simulink model "HANcoder_E407_GTSync_v5"  (R2018b)
settings: Solver=FixedStepDiscrete  StartTime=0.0  StopTime=1  FixedStep=0.01  RelTol=1e-3
PreLoadFcn:
  | librarySetup
  | eval([bdroot,'_startup']) %Calling [modelName]_startup.m
values from neighbouring files (symbols this model uses):
  basic_cycle_duration = TM_Reset_Board + COMP_duration    (= 170)    [HANcoder_E407_GTSync_v5_startup.m]
  comm_delay_estimation1 = round(comm_delay_measured*hardware_granularity/frequency_IRQ)    [HANcoder_E407_GTSync_v5_startup.m]
  comm_delay_estimation2 = round(comm_delay_measured*hardware_granularity/frequency_IRQ)    [HANcoder_E407_GTSync_v5_startup.m]
  COMM_Period = 25    [HANcoder_E407_GTSync_v5_startup.m]
  COMM_Phase1 = floor(COMM_Period/5)    [HANcoder_E407_GTSync_v5_startup.m]
  COMM_Phase2 = floor(4*COMM_Period/5)    [HANcoder_E407_GTSync_v5_startup.m]
  frequency_IRQ = 100    [HANcoder_E407_GTSync_v5_startup.m]
  HANtuneOverride = Simulink.Parameter    [HANcoder_E407_GTSync_v5_startup.m]
  idle_time_init = basic_cycle_duration*matrix_rows    (= 340)    [HANcoder_E407_GTSync_v5_startup.m]
  LED_ticks_toggle = 10000    [HANcoder_E407_GTSync_v5_startup.m]
  Master_Role = 1    [HANcoder_E407_GTSync_v5_startup.m]
  matrix_rows = 2    [HANcoder_E407_GTSync_v5_startup.m]
  MEX_Flag = 0    [HANcoder_E407_GTSync_v5_startup.m]
  Slave_Role = 2    [HANcoder_E407_GTSync_v5_startup.m]
  Sync_ID = 1    [HANcoder_E407_GTSync_v5_startup.m]
  TM_Check_Sync = TM_COMM_Sync   + COMM_duration    (= 30)    [HANcoder_E407_GTSync_v5_startup.m]
  TM_Check_TOuts = TM_Count_Vote3 + COMP_duration    (= 150)    [HANcoder_E407_GTSync_v5_startup.m]
  TM_Check_Vote1 = TM_COMM_Vote1  + COMM_duration    (= 70)    [HANcoder_E407_GTSync_v5_startup.m]
  TM_Check_Vote2 = TM_COMM_Vote2  + COMM_duration    (= 105)    [HANcoder_E407_GTSync_v5_startup.m]
  TM_Check_Vote3 = TM_COMM_Vote3  + COMM_duration    (= 140)    [HANcoder_E407_GTSync_v5_startup.m]
  TM_COMM_Sync = basic_cycle_start    (= 5)    [HANcoder_E407_GTSync_v5_startup.m]
  TM_COMM_Vote1 = TM_Vote_Dec    + COMP_duration    (= 45)    [HANcoder_E407_GTSync_v5_startup.m]
  TM_COMM_Vote2 = TM_Count_Vote1 + COMP_duration    (= 80)    [HANcoder_E407_GTSync_v5_startup.m]
  TM_COMM_Vote3 = TM_Count_Vote2 + COMP_duration    (= 115)    [HANcoder_E407_GTSync_v5_startup.m]
  TM_Count_Vote1 = TM_Check_Vote1 + COMP_duration    (= 75)    [HANcoder_E407_GTSync_v5_startup.m]
  TM_Count_Vote2 = TM_Check_Vote2 + COMP_duration    (= 110)    [HANcoder_E407_GTSync_v5_startup.m]
  TM_Count_Vote3 = TM_Check_Vote3 + COMP_duration    (= 145)    [HANcoder_E407_GTSync_v5_startup.m]
  TM_New_Master = TM_Check_TOuts + COMP_duration    (= 155)    [HANcoder_E407_GTSync_v5_startup.m]
  TM_Reset_Board = TM_Reset_Var   + COMP_duration    (= 165)    [HANcoder_E407_GTSync_v5_startup.m]
  TM_Reset_Var = TM_New_Master  + COMP_duration    (= 160)    [HANcoder_E407_GTSync_v5_startup.m]
  TM_Update_LT = TM_Check_Sync  + COMP_duration    (= 35)    [HANcoder_E407_GTSync_v5_startup.m]
  TM_Vote_Dec = TM_Update_LT   + COMP_duration    (= 40)    [HANcoder_E407_GTSync_v5_startup.m]
  Toggle_Flag = 1    [HANcoder_E407_GTSync_v5_startup.m]
  Vote1_ID = 12    [HANcoder_E407_GTSync_v5_startup.m]
  Vote2_ID = 22    [HANcoder_E407_GTSync_v5_startup.m]
  Vote3_ID = 32    [HANcoder_E407_GTSync_v5_startup.m]
undefined symbols (not defined in the file or in its folder): A0, A1, A2, A3, CON2
libraries: HANcoder_STM32_Target x25, hdlsllib x21, simulink x3, simulink_extras x1
(part 7 of 7)

== system HANcoder_E407_GTSync_v5/HANcoder STM32 Target - E407-STM32 algorithm/Global Ticks Increment/CAN Management/Matrix Cycle Manager/COMP Task - Rx_Vote2_Check/Process_Messages1/Demux message CAN1 and check coherence ==
  CAN1_Rx_msg : Inport  OutDataTypeStr=Bus: msg_buffer_type
  expected_local_time : Inport  Port=2
  expected_basic_cycle : Inport  Port=3
  Enable : EnablePort
  AND : Logic  IconShape=distinctive  AllPortsSameDT=off  OutDataTypeStr=boolean
  Bus Creator : BusCreator  Inputs=3  OutDataTypeStr=Bus: demux_msg_buffer_type
  Bus Selector : BusSelector  OutputSignals=Buffer_1,Buffer_2,Buffer_3,Buffer_4,Buffer_5,Buffer_6,Buffer_7,Buffer_8
  Equal : RelationalOperator  Operator===  OutDataTypeStr=boolean  RndMeth=Simplest
  Equal2 : RelationalOperator  Operator===  OutDataTypeStr=boolean  RndMeth=Simplest
  Terminator{3..4,6..7} (4 alike) : Terminator
  UINT8 to UINT16 : Subsystem
  CAN1_msg : Outport  OutDataTypeStr=Bus: demux_msg_buffer_type
  CAN1_msg_coherent : Outport  Port=2  OutputWhenDisabled=reset  InitialOutput=0
  wires:
  Bus Selector/2 -> UINT8 to UINT16/1(In1)  "<Buffer_2>"
  UINT8 to UINT16/1(Out1) -> Bus Creator/2, Equal/1
  Bus Selector/1 -> Bus Creator/1  "<Buffer_1>"
  Bus Selector/4 -> Bus Creator/3, Equal2/1  "<Buffer_4>"
  Bus Selector/3 -> UINT8 to UINT16/2(In2)  "<Buffer_3>"
  CAN1_Rx_msg/1 -> Bus Selector/1
  Equal2/1 -> AND/2
  Equal/1 -> AND/1
  AND/1 -> CAN1_msg_coherent/1
  expected_local_time/1 -> Equal/2
  expected_basic_cycle/1 -> Equal2/2
  Bus Creator/1 -> CAN1_msg/1
  Bus Selector/6 -> Terminator3/1  "<Buffer_6>"
  Bus Selector/5 -> Terminator4/1  "<Buffer_5>"
  Bus Selector/7 -> Terminator6/1  "<Buffer_7>"
  Bus Selector/8 -> Terminator7/1  "<Buffer_8>"

== system HANcoder_E407_GTSync_v5/HANcoder STM32 Target - E407-STM32 algorithm/Global Ticks Increment/CAN Management/Matrix Cycle Manager/COMP Task - Rx_Vote2_Check/Process_Messages1/Demux message CAN2 and check coherence ==
  CAN2_Rx_msg : Inport  OutDataTypeStr=Bus: msg_buffer_type
  expected_local_time : Inport  Port=2
  expected_basic_cycle : Inport  Port=3
  Enable : EnablePort
  AND : Logic  IconShape=distinctive  AllPortsSameDT=off  OutDataTypeStr=boolean
  Bus Creator : BusCreator  Inputs=3  OutDataTypeStr=Bus: demux_msg_buffer_type
  Bus Selector : BusSelector  OutputSignals=Buffer_1,Buffer_2,Buffer_3,Buffer_4,Buffer_5,Buffer_6,Buffer_7,Buffer_8
  Equal : RelationalOperator  Operator===  OutDataTypeStr=boolean  RndMeth=Simplest
  Equal2 : RelationalOperator  Operator===  OutDataTypeStr=boolean  RndMeth=Simplest
  Terminator{3..4,6..7} (4 alike) : Terminator
  UINT8 to UINT16 : Subsystem
  CAN2_msg_coherent : Outport  OutputWhenDisabled=reset  InitialOutput=0
  CAN2_msg : Outport  Port=2  OutDataTypeStr=Bus: demux_msg_buffer_type
  wires:
  Bus Selector/2 -> UINT8 to UINT16/1(In1)  "<Buffer_2>"
  UINT8 to UINT16/1(Out1) -> Bus Creator/2, Equal/1
  Bus Selector/1 -> Bus Creator/1  "<Buffer_1>"
  Bus Selector/4 -> Bus Creator/3, Equal2/1  "<Buffer_4>"
  Bus Selector/3 -> UINT8 to UINT16/2(In2)  "<Buffer_3>"
  CAN2_Rx_msg/1 -> Bus Selector/1
  Equal/1 -> AND/1  "expected_lt_Vote2_CAN2_s"
  AND/1 -> CAN2_msg_coherent/1
  expected_local_time/1 -> Equal/2
  expected_basic_cycle/1 -> Equal2/2
  Bus Creator/1 -> CAN2_msg/1
  Bus Selector/6 -> Terminator3/1  "<Buffer_6>"
  Bus Selector/5 -> Terminator4/1  "<Buffer_5>"
  Bus Selector/7 -> Terminator6/1  "<Buffer_7>"
  Bus Selector/8 -> Terminator7/1  "<Buffer_8>"
  Equal2/1 -> AND/2  "expected_bc_Vote2_CAN2_s"

== system HANcoder_E407_GTSync_v5/HANcoder STM32 Target - E407-STM32 algorithm/Global Ticks Increment/CAN Management/Matrix Cycle Manager/COMP Task - Rx_Vote3_Check/Process_Messages1/Demux message CAN1 and check coherence ==
  CAN1_Rx_msg : Inport  OutDataTypeStr=Bus: msg_buffer_type
  expected_local_time : Inport  Port=2
  expected_basic_cycle : Inport  Port=3
  Enable : EnablePort
  AND : Logic  IconShape=distinctive  AllPortsSameDT=off  OutDataTypeStr=boolean
  Bus Creator : BusCreator  Inputs=3  OutDataTypeStr=Bus: demux_msg_buffer_type
  Bus Selector : BusSelector  OutputSignals=Buffer_1,Buffer_2,Buffer_3,Buffer_4,Buffer_5,Buffer_6,Buffer_7,Buffer_8
  Equal : RelationalOperator  Operator===  OutDataTypeStr=boolean  RndMeth=Simplest
  Equal2 : RelationalOperator  Operator===  OutDataTypeStr=boolean  RndMeth=Simplest
  Terminator{3..4,6..7} (4 alike) : Terminator
  UINT8 to UINT16 : Subsystem
  CAN1_msg : Outport  OutDataTypeStr=Bus: demux_msg_buffer_type
  CAN1_msg_coherent : Outport  Port=2  OutputWhenDisabled=reset  InitialOutput=0
  wires:
  Bus Selector/2 -> UINT8 to UINT16/1(In1)  "<Buffer_2>"
  UINT8 to UINT16/1(Out1) -> Bus Creator/2, Equal/1
  Bus Selector/1 -> Bus Creator/1  "<Buffer_1>"
  Bus Selector/4 -> Bus Creator/3, Equal2/1  "<Buffer_4>"
  Bus Selector/3 -> UINT8 to UINT16/2(In2)  "<Buffer_3>"
  CAN1_Rx_msg/1 -> Bus Selector/1
  AND/1 -> CAN1_msg_coherent/1
  expected_local_time/1 -> Equal/2
  expected_basic_cycle/1 -> Equal2/2
  Bus Creator/1 -> CAN1_msg/1
  Bus Selector/6 -> Terminator3/1  "<Buffer_6>"
  Bus Selector/5 -> Terminator4/1  "<Buffer_5>"
  Bus Selector/7 -> Terminator6/1  "<Buffer_7>"
  Bus Selector/8 -> Terminator7/1  "<Buffer_8>"
  Equal/1 -> AND/1
  Equal2/1 -> AND/2

== system HANcoder_E407_GTSync_v5/HANcoder STM32 Target - E407-STM32 algorithm/Global Ticks Increment/CAN Management/Matrix Cycle Manager/COMP Task - Rx_Vote3_Check/Process_Messages1/Demux message CAN2 and check coherence ==
  CAN2_Rx_msg : Inport  OutDataTypeStr=Bus: msg_buffer_type
  expected_local_time : Inport  Port=2
  expected_basic_cycle : Inport  Port=3
  Enable : EnablePort
  AND : Logic  IconShape=distinctive  AllPortsSameDT=off  OutDataTypeStr=boolean
  Bus Creator : BusCreator  Inputs=3  OutDataTypeStr=Bus: demux_msg_buffer_type
  Bus Selector : BusSelector  OutputSignals=Buffer_1,Buffer_2,Buffer_3,Buffer_4,Buffer_5,Buffer_6,Buffer_7,Buffer_8
  Equal : RelationalOperator  Operator===  OutDataTypeStr=boolean  RndMeth=Simplest
  Equal2 : RelationalOperator  Operator===  OutDataTypeStr=boolean  RndMeth=Simplest
  Terminator{3..4,6..7} (4 alike) : Terminator
  UINT8 to UINT16 : Subsystem
  CAN2_msg_coherent : Outport  OutputWhenDisabled=reset  InitialOutput=0
  CAN2_msg : Outport  Port=2  OutDataTypeStr=Bus: demux_msg_buffer_type
  wires:
  Bus Selector/2 -> UINT8 to UINT16/1(In1)  "<Buffer_2>"
  UINT8 to UINT16/1(Out1) -> Bus Creator/2, Equal/1
  Bus Selector/1 -> Bus Creator/1  "<Buffer_1>"
  Bus Selector/4 -> Bus Creator/3, Equal2/1  "<Buffer_4>"
  Bus Selector/3 -> UINT8 to UINT16/2(In2)  "<Buffer_3>"
  CAN2_Rx_msg/1 -> Bus Selector/1
  AND/1 -> CAN2_msg_coherent/1
  expected_local_time/1 -> Equal/2
  expected_basic_cycle/1 -> Equal2/2
  Bus Creator/1 -> CAN2_msg/1
  Bus Selector/6 -> Terminator3/1  "<Buffer_6>"
  Bus Selector/5 -> Terminator4/1  "<Buffer_5>"
  Bus Selector/7 -> Terminator6/1  "<Buffer_7>"
  Bus Selector/8 -> Terminator7/1  "<Buffer_8>"
  Equal/1 -> AND/1  "expected_lt_Vote3_CAN2_s"
  Equal2/1 -> AND/2  "expected_bc_Vote3_CAN2_s"

== system HANcoder_E407_GTSync_v5/HANcoder STM32 Target - E407-STM32 algorithm/Global Ticks Increment/CAN Management/Matrix Cycle Manager/COMP Task - Update LT/Local Time Update/Desync_Negative ==
  note: Local time correction when Desync is negative
      | In this case the Local Time "goes back in time".
      | Previous tasks will not be activated because
      | sync_processed flag is alread set.
  note: Current Local Time correction
  note: Local Time Update
  Enable : EnablePort
  Cast : DataTypeConversion  Priority=13  OutDataTypeStr=uint16
  Current_local_time : Constant  Priority=10  Value=TM_Update_LT  OutDataTypeStr=uint16
  Data Store Read : DataStoreRead  Priority=11  DataStoreName=Desync_Ticks
  Data Store Write1 : DataStoreWrite  Priority=14  DataStoreName=Local_Ticks  DataStoreElements=Local_Ticks
  Minus : Sum  Priority=12
  wires:
  Data Store Read/1 -> Minus/2
  Minus/1 -> Cast/1  "RX_LT_Master_bc0_s"
  Cast/1 -> Data Store Write1/1
  Current_local_time/1 -> Minus/1

== system HANcoder_E407_GTSync_v5/HANcoder STM32 Target - E407-STM32 algorithm/Global Ticks Increment/CAN Management/Matrix Cycle Manager/COMP Task - Vote Decision/Vote Decision/Ensure no self votes or failed master reelected ==
  Node ID : Inport
  Sync Timeout : Inport  Port=2
  Error counter : Inport  Port=3
  AND : Logic  IconShape=distinctive  AllPortsSameDT=off  OutDataTypeStr=boolean
  Data Store Read : DataStoreRead  DataStoreName=Board_ID
  Data Store Read2 : DataStoreRead  DataStoreName=Master_ID
  Equal1 : RelationalOperator  Operator===  OutDataTypeStr=boolean  RndMeth=Simplest
  Equal2 : RelationalOperator  Operator===  OutDataTypeStr=boolean  RndMeth=Simplest
  MAX error count : Constant  Value=4294967295  OutDataTypeStr=uint32
  NOT : Logic  Operator=NOT  IconShape=distinctive  AllPortsSameDT=off  OutDataTypeStr=boolean
  OR : Logic  Operator=OR  IconShape=distinctive  AllPortsSameDT=off  OutDataTypeStr=boolean
  Switch : Switch  Criteria=u2 > Threshold
  Out1 : Outport
  wires:
  Equal1/1 -> OR/1
  Data Store Read/1 -> Equal1/2
  MAX error count/1 -> Switch/1
  Switch/1 -> Out1/1
  Error counter/1 -> Switch/3
  Node ID/1 -> Equal1/1, Equal2/2
  Sync Timeout/1 -> NOT/1
  Data Store Read2/1 -> Equal2/1
  Equal2/1 -> AND/1
  NOT/1 -> AND/2
  AND/1 -> OR/2
  OR/1 -> Switch/2

== system HANcoder_E407_GTSync_v5/HANcoder STM32 Target - E407-STM32 algorithm/Global Ticks Increment/CAN Management/Matrix Cycle Manager/COMP Task - Vote Decision/Vote Decision/Ensure no self votes or failed master reelected1 ==
  Node ID : Inport
  Sync Timeout : Inport  Port=2
  Error counter : Inport  Port=3
  AND : Logic  IconShape=distinctive  AllPortsSameDT=off  OutDataTypeStr=boolean
  Data Store Read : DataStoreRead  DataStoreName=Board_ID
  Data Store Read2 : DataStoreRead  DataStoreName=Master_ID
  Equal1 : RelationalOperator  Operator===  OutDataTypeStr=boolean  RndMeth=Simplest
  Equal2 : RelationalOperator  Operator===  OutDataTypeStr=boolean  RndMeth=Simplest
  MAX error count : Constant  Value=4294967295  OutDataTypeStr=uint32
  NOT : Logic  Operator=NOT  IconShape=distinctive  AllPortsSameDT=off  OutDataTypeStr=boolean
  OR : Logic  Operator=OR  IconShape=distinctive  AllPortsSameDT=off  OutDataTypeStr=boolean
  Switch : Switch  Criteria=u2 > Threshold
  Out1 : Outport
  wires:
  OR/1 -> Switch/2
  AND/1 -> OR/2
  NOT/1 -> AND/2
  Equal2/1 -> AND/1
  Data Store Read2/1 -> Equal2/1
  Sync Timeout/1 -> NOT/1
  Node ID/1 -> Equal2/2, Equal1/1
  Error counter/1 -> Switch/3
  Switch/1 -> Out1/1
  MAX error count/1 -> Switch/1
  Data Store Read/1 -> Equal1/2
  Equal1/1 -> OR/1

== system HANcoder_E407_GTSync_v5/HANcoder STM32 Target - E407-STM32 algorithm/Global Ticks Increment/CAN Management/Matrix Cycle Manager/COMP Task - Vote Decision/Vote Decision/Ensure no self votes or failed master reelected2 ==
  Node ID : Inport
  Sync Timeout : Inport  Port=2
  Error counter : Inport  Port=3
  AND : Logic  IconShape=distinctive  AllPortsSameDT=off  OutDataTypeStr=boolean
  Data Store Read : DataStoreRead  DataStoreName=Board_ID
  Data Store Read2 : DataStoreRead  DataStoreName=Master_ID
  Equal1 : RelationalOperator  Operator===  OutDataTypeStr=boolean  RndMeth=Simplest
  Equal2 : RelationalOperator  Operator===  OutDataTypeStr=boolean  RndMeth=Simplest
  MAX error count : Constant  Value=4294967295  OutDataTypeStr=uint32
  NOT : Logic  Operator=NOT  IconShape=distinctive  AllPortsSameDT=off  OutDataTypeStr=boolean
  OR : Logic  Operator=OR  IconShape=distinctive  AllPortsSameDT=off  OutDataTypeStr=boolean
  Switch : Switch  Criteria=u2 > Threshold
  Out1 : Outport
  wires:
  Equal1/1 -> OR/1
  Data Store Read/1 -> Equal1/2
  MAX error count/1 -> Switch/1
  Switch/1 -> Out1/1
  Error counter/1 -> Switch/3
  Node ID/1 -> Equal1/1, Equal2/2
  Sync Timeout/1 -> NOT/1
  Data Store Read2/1 -> Equal2/1
  Equal2/1 -> AND/1
  NOT/1 -> AND/2
  AND/1 -> OR/2
  OR/1 -> Switch/2

== system HANcoder_E407_GTSync_v5/HANcoder STM32 Target - E407-STM32 algorithm/Global Ticks Increment/CAN1 Recieve/RxID_CAN/Sync_ID_CAN/CAN receive/Enabled Subsystem ==
  In1 : Inport
  In2 : Inport  Port=2
  In3 : Inport  Port=3
  In4 : Inport  Port=4
  In5 : Inport  Port=5
  In6 : Inport  Port=6
  In7 : Inport  Port=7
  In8 : Inport  Port=8
  Enable : EnablePort
  Out1 : Outport
  Out2 : Outport  Port=2
  Out3 : Outport  Port=3
  Out4 : Outport  Port=4
  Out5 : Outport  Port=5
  Out6 : Outport  Port=6
  Out7 : Outport  Port=7
  Out8 : Outport  Port=8
  wires:
  In8/1 -> Out8/1
  In7/1 -> Out7/1
  In6/1 -> Out6/1
  In5/1 -> Out5/1
  In4/1 -> Out4/1
  In3/1 -> Out3/1
  In2/1 -> Out2/1
  In1/1 -> Out1/1

== system HANcoder_E407_GTSync_v5/HANcoder STM32 Target - E407-STM32 algorithm/Global Ticks Increment/CAN1 Recieve/RxID_CAN/Vote1_ID_CAN/CAN receive/Enabled Subsystem ==
  In1 : Inport
  In2 : Inport  Port=2
  In3 : Inport  Port=3
  In4 : Inport  Port=4
  In5 : Inport  Port=5
  In6 : Inport  Port=6
  In7 : Inport  Port=7
  In8 : Inport  Port=8
  Enable : EnablePort
  Out1 : Outport
  Out2 : Outport  Port=2
  Out3 : Outport  Port=3
  Out4 : Outport  Port=4
  Out5 : Outport  Port=5
  Out6 : Outport  Port=6
  Out7 : Outport  Port=7
  Out8 : Outport  Port=8
  wires:
  In1/1 -> Out1/1
  In2/1 -> Out2/1
  In3/1 -> Out3/1
  In4/1 -> Out4/1
  In5/1 -> Out5/1
  In6/1 -> Out6/1
  In7/1 -> Out7/1
  In8/1 -> Out8/1

== system HANcoder_E407_GTSync_v5/HANcoder STM32 Target - E407-STM32 algorithm/Global Ticks Increment/CAN1 Recieve/RxID_CAN/Vote2_ID_CAN/CAN receive/Enabled Subsystem ==
  In1 : Inport
  In2 : Inport  Port=2
  In3 : Inport  Port=3
  In4 : Inport  Port=4
  In5 : Inport  Port=5
  In6 : Inport  Port=6
  In7 : Inport  Port=7
  In8 : Inport  Port=8
  Enable : EnablePort
  Out1 : Outport
  Out2 : Outport  Port=2
  Out3 : Outport  Port=3
  Out4 : Outport  Port=4
  Out5 : Outport  Port=5
  Out6 : Outport  Port=6
  Out7 : Outport  Port=7
  Out8 : Outport  Port=8
  wires:
  In8/1 -> Out8/1
  In7/1 -> Out7/1
  In6/1 -> Out6/1
  In5/1 -> Out5/1
  In4/1 -> Out4/1
  In3/1 -> Out3/1
  In2/1 -> Out2/1
  In1/1 -> Out1/1

== system HANcoder_E407_GTSync_v5/HANcoder STM32 Target - E407-STM32 algorithm/Global Ticks Increment/CAN1 Recieve/RxID_CAN/Vote3_ID_CAN/CAN receive/Enabled Subsystem ==
  In1 : Inport
  In2 : Inport  Port=2
  In3 : Inport  Port=3
  In4 : Inport  Port=4
  In5 : Inport  Port=5
  In6 : Inport  Port=6
  In7 : Inport  Port=7
  In8 : Inport  Port=8
  Enable : EnablePort
  Out1 : Outport
  Out2 : Outport  Port=2
  Out3 : Outport  Port=3
  Out4 : Outport  Port=4
  Out5 : Outport  Port=5
  Out6 : Outport  Port=6
  Out7 : Outport  Port=7
  Out8 : Outport  Port=8
  wires:
  In1/1 -> Out1/1
  In2/1 -> Out2/1
  In3/1 -> Out3/1
  In4/1 -> Out4/1
  In5/1 -> Out5/1
  In6/1 -> Out6/1
  In7/1 -> Out7/1
  In8/1 -> Out8/1

== system HANcoder_E407_GTSync_v5/HANcoder STM32 Target - E407-STM32 algorithm/Global Ticks Increment/CAN2 Recieve/RxID_CAN/Sync_ID_CAN/CAN receive/Enabled Subsystem ==
  In1 : Inport
  In2 : Inport  Port=2
  In3 : Inport  Port=3
  In4 : Inport  Port=4
  In5 : Inport  Port=5
  In6 : Inport  Port=6
  In7 : Inport  Port=7
  In8 : Inport  Port=8
  Enable : EnablePort
  Out1 : Outport
  Out2 : Outport  Port=2
  Out3 : Outport  Port=3
  Out4 : Outport  Port=4
  Out5 : Outport  Port=5
  Out6 : Outport  Port=6
  Out7 : Outport  Port=7
  Out8 : Outport  Port=8
  wires:
  In1/1 -> Out1/1
  In2/1 -> Out2/1
  In3/1 -> Out3/1
  In4/1 -> Out4/1
  In5/1 -> Out5/1
  In6/1 -> Out6/1
  In7/1 -> Out7/1
  In8/1 -> Out8/1

== system HANcoder_E407_GTSync_v5/HANcoder STM32 Target - E407-STM32 algorithm/Global Ticks Increment/CAN2 Recieve/RxID_CAN/Vote1_ID_CAN/CAN receive/Enabled Subsystem ==
  In1 : Inport
  In2 : Inport  Port=2
  In3 : Inport  Port=3
  In4 : Inport  Port=4
  In5 : Inport  Port=5
  In6 : Inport  Port=6
  In7 : Inport  Port=7
  In8 : Inport  Port=8
  Enable : EnablePort
  Out1 : Outport
  Out2 : Outport  Port=2
  Out3 : Outport  Port=3
  Out4 : Outport  Port=4
  Out5 : Outport  Port=5
  Out6 : Outport  Port=6
  Out7 : Outport  Port=7
  Out8 : Outport  Port=8
  wires:
  In8/1 -> Out8/1
  In7/1 -> Out7/1
  In6/1 -> Out6/1
  In5/1 -> Out5/1
  In4/1 -> Out4/1
  In3/1 -> Out3/1
  In2/1 -> Out2/1
  In1/1 -> Out1/1

== system HANcoder_E407_GTSync_v5/HANcoder STM32 Target - E407-STM32 algorithm/Global Ticks Increment/CAN2 Recieve/RxID_CAN/Vote2_ID_CAN/CAN receive/Enabled Subsystem ==
  In1 : Inport
  In2 : Inport  Port=2
  In3 : Inport  Port=3
  In4 : Inport  Port=4
  In5 : Inport  Port=5
  In6 : Inport  Port=6
  In7 : Inport  Port=7
  In8 : Inport  Port=8
  Enable : EnablePort
  Out1 : Outport
  Out2 : Outport  Port=2
  Out3 : Outport  Port=3
  Out4 : Outport  Port=4
  Out5 : Outport  Port=5
  Out6 : Outport  Port=6
  Out7 : Outport  Port=7
  Out8 : Outport  Port=8
  wires:
  In1/1 -> Out1/1
  In2/1 -> Out2/1
  In3/1 -> Out3/1
  In4/1 -> Out4/1
  In5/1 -> Out5/1
  In6/1 -> Out6/1
  In7/1 -> Out7/1
  In8/1 -> Out8/1

== system HANcoder_E407_GTSync_v5/HANcoder STM32 Target - E407-STM32 algorithm/Global Ticks Increment/CAN2 Recieve/RxID_CAN/Vote3_ID_CAN/CAN receive/Enabled Subsystem ==
  In1 : Inport
  In2 : Inport  Port=2
  In3 : Inport  Port=3
  In4 : Inport  Port=4
  In5 : Inport  Port=5
  In6 : Inport  Port=6
  In7 : Inport  Port=7
  In8 : Inport  Port=8
  Enable : EnablePort
  Out1 : Outport
  Out2 : Outport  Port=2
  Out3 : Outport  Port=3
  Out4 : Outport  Port=4
  Out5 : Outport  Port=5
  Out6 : Outport  Port=6
  Out7 : Outport  Port=7
  Out8 : Outport  Port=8
  wires:
  In8/1 -> Out8/1
  In7/1 -> Out7/1
  In6/1 -> Out6/1
  In5/1 -> Out5/1
  In4/1 -> Out4/1
  In3/1 -> Out3/1
  In2/1 -> Out2/1
  In1/1 -> Out1/1

== system HANcoder_E407_GTSync_v5/HANcoder STM32 Target - E407-STM32 algorithm/Global Ticks Increment/CAN Management/Matrix Cycle Manager/COMP Task - Rx_Sync_Check/Process_Messages/Demux message CAN1 and check coherence/UINT8 to UINT16 ==
  In1 : Inport
  In2 : Inport  Port=2
  Bit Shift : hdlsllib/Logic and Bit Operations/Bit Shift  mode=Shift Left Logical  N=8
      settings: SourceProductName=HDL Coder  SourceProductBaseCode=HD
  Cast1 : DataTypeConversion  OutDataTypeStr=uint16
  Cast4 : DataTypeConversion  OutDataTypeStr=uint16
  Sum1 : Sum
  Out1 : Outport
  wires:
  Cast4/1 -> Sum1/1
  Sum1/1 -> Out1/1
  In2/1 -> Cast1/1
  Cast1/1 -> Bit Shift/1
  Bit Shift/1 -> Sum1/2
  In1/1 -> Cast4/1

== system HANcoder_E407_GTSync_v5/HANcoder STM32 Target - E407-STM32 algorithm/Global Ticks Increment/CAN Management/Matrix Cycle Manager/COMP Task - Rx_Sync_Check/Process_Messages/Demux message CAN2 and check coherence/UINT8 to UINT16 ==
  In1 : Inport
  In2 : Inport  Port=2
  Bit Shift : hdlsllib/Logic and Bit Operations/Bit Shift  mode=Shift Left Logical  N=8
      settings: SourceProductName=HDL Coder  SourceProductBaseCode=HD
  Cast1 : DataTypeConversion  OutDataTypeStr=uint16
  Cast4 : DataTypeConversion  OutDataTypeStr=uint16
  Sum1 : Sum
  Out1 : Outport
  wires:
  Cast4/1 -> Sum1/1
  Sum1/1 -> Out1/1
  In2/1 -> Cast1/1
  Cast1/1 -> Bit Shift/1
  Bit Shift/1 -> Sum1/2
  In1/1 -> Cast4/1

== system HANcoder_E407_GTSync_v5/HANcoder STM32 Target - E407-STM32 algorithm/Global Ticks Increment/CAN Management/Matrix Cycle Manager/COMP Task - Rx_Sync_Check - bc1/Process_Messages/Demux message CAN1 and check coherence/UINT8 to UINT16 ==
  In1 : Inport
  In2 : Inport  Port=2
  Bit Shift : hdlsllib/Logic and Bit Operations/Bit Shift  mode=Shift Left Logical  N=8
      settings: SourceProductName=HDL Coder  SourceProductBaseCode=HD
  Cast1 : DataTypeConversion  OutDataTypeStr=uint16
  Cast4 : DataTypeConversion  OutDataTypeStr=uint16
  Sum1 : Sum
  Out1 : Outport
  wires:
  Cast4/1 -> Sum1/1
  Sum1/1 -> Out1/1
  In2/1 -> Cast1/1
  Cast1/1 -> Bit Shift/1
  Bit Shift/1 -> Sum1/2
  In1/1 -> Cast4/1

== system HANcoder_E407_GTSync_v5/HANcoder STM32 Target - E407-STM32 algorithm/Global Ticks Increment/CAN Management/Matrix Cycle Manager/COMP Task - Rx_Sync_Check - bc1/Process_Messages/Demux message CAN2 and check coherence/UINT8 to UINT16 ==
  In1 : Inport
  In2 : Inport  Port=2
  Bit Shift : hdlsllib/Logic and Bit Operations/Bit Shift  mode=Shift Left Logical  N=8
      settings: SourceProductName=HDL Coder  SourceProductBaseCode=HD
  Cast1 : DataTypeConversion  OutDataTypeStr=uint16
  Cast4 : DataTypeConversion  OutDataTypeStr=uint16
  Sum1 : Sum
  Out1 : Outport
  wires:
  Cast4/1 -> Sum1/1
  Sum1/1 -> Out1/1
  In2/1 -> Cast1/1
  Cast1/1 -> Bit Shift/1
  Bit Shift/1 -> Sum1/2
  In1/1 -> Cast4/1

== system HANcoder_E407_GTSync_v5/HANcoder STM32 Target - E407-STM32 algorithm/Global Ticks Increment/CAN Management/Matrix Cycle Manager/COMP Task - Rx_Vote1_Check/Process_Messages1/Demux message CAN1 and check coherence/UINT8 to UINT16 ==
  In1 : Inport
  In2 : Inport  Port=2
  Bit Shift : hdlsllib/Logic and Bit Operations/Bit Shift  mode=Shift Left Logical  N=8
      settings: SourceProductName=HDL Coder  SourceProductBaseCode=HD
  Cast1 : DataTypeConversion  OutDataTypeStr=uint16
  Cast4 : DataTypeConversion  OutDataTypeStr=uint16
  Sum1 : Sum
  Out1 : Outport
  wires:
  Cast4/1 -> Sum1/1
  Sum1/1 -> Out1/1
  In2/1 -> Cast1/1
  Cast1/1 -> Bit Shift/1
  Bit Shift/1 -> Sum1/2
  In1/1 -> Cast4/1

== system HANcoder_E407_GTSync_v5/HANcoder STM32 Target - E407-STM32 algorithm/Global Ticks Increment/CAN Management/Matrix Cycle Manager/COMP Task - Rx_Vote1_Check/Process_Messages1/Demux message CAN2 and check coherence/UINT8 to UINT16 ==
  In1 : Inport
  In2 : Inport  Port=2
  Bit Shift : hdlsllib/Logic and Bit Operations/Bit Shift  mode=Shift Left Logical  N=8
      settings: SourceProductName=HDL Coder  SourceProductBaseCode=HD
  Cast1 : DataTypeConversion  OutDataTypeStr=uint16
  Cast4 : DataTypeConversion  OutDataTypeStr=uint16
  Sum1 : Sum
  Out1 : Outport
  wires:
  Cast4/1 -> Sum1/1
  Sum1/1 -> Out1/1
  In2/1 -> Cast1/1
  Cast1/1 -> Bit Shift/1
  Bit Shift/1 -> Sum1/2
  In1/1 -> Cast4/1

== system HANcoder_E407_GTSync_v5/HANcoder STM32 Target - E407-STM32 algorithm/Global Ticks Increment/CAN Management/Matrix Cycle Manager/COMP Task - Rx_Vote2_Check/Process_Messages1/Demux message CAN1 and check coherence/UINT8 to UINT16 ==
  In1 : Inport
  In2 : Inport  Port=2
  Bit Shift : hdlsllib/Logic and Bit Operations/Bit Shift  mode=Shift Left Logical  N=8
      settings: SourceProductName=HDL Coder  SourceProductBaseCode=HD
  Cast1 : DataTypeConversion  OutDataTypeStr=uint16
  Cast4 : DataTypeConversion  OutDataTypeStr=uint16
  Sum1 : Sum
  Out1 : Outport
  wires:
  Cast4/1 -> Sum1/1
  Sum1/1 -> Out1/1
  In2/1 -> Cast1/1
  Cast1/1 -> Bit Shift/1
  Bit Shift/1 -> Sum1/2
  In1/1 -> Cast4/1

== system HANcoder_E407_GTSync_v5/HANcoder STM32 Target - E407-STM32 algorithm/Global Ticks Increment/CAN Management/Matrix Cycle Manager/COMP Task - Rx_Vote2_Check/Process_Messages1/Demux message CAN2 and check coherence/UINT8 to UINT16 ==
  In1 : Inport
  In2 : Inport  Port=2
  Bit Shift : hdlsllib/Logic and Bit Operations/Bit Shift  mode=Shift Left Logical  N=8
      settings: SourceProductName=HDL Coder  SourceProductBaseCode=HD
  Cast1 : DataTypeConversion  OutDataTypeStr=uint16
  Cast4 : DataTypeConversion  OutDataTypeStr=uint16
  Sum1 : Sum
  Out1 : Outport
  wires:
  Cast4/1 -> Sum1/1
  Sum1/1 -> Out1/1
  In2/1 -> Cast1/1
  Cast1/1 -> Bit Shift/1
  Bit Shift/1 -> Sum1/2
  In1/1 -> Cast4/1

== system HANcoder_E407_GTSync_v5/HANcoder STM32 Target - E407-STM32 algorithm/Global Ticks Increment/CAN Management/Matrix Cycle Manager/COMP Task - Rx_Vote3_Check/Process_Messages1/Demux message CAN1 and check coherence/UINT8 to UINT16 ==
  In1 : Inport
  In2 : Inport  Port=2
  Bit Shift : hdlsllib/Logic and Bit Operations/Bit Shift  mode=Shift Left Logical  N=8
      settings: SourceProductName=HDL Coder  SourceProductBaseCode=HD
  Cast1 : DataTypeConversion  OutDataTypeStr=uint16
  Cast4 : DataTypeConversion  OutDataTypeStr=uint16
  Sum1 : Sum
  Out1 : Outport
  wires:
  Cast4/1 -> Sum1/1
  Sum1/1 -> Out1/1
  In2/1 -> Cast1/1
  Cast1/1 -> Bit Shift/1
  Bit Shift/1 -> Sum1/2
  In1/1 -> Cast4/1

== system HANcoder_E407_GTSync_v5/HANcoder STM32 Target - E407-STM32 algorithm/Global Ticks Increment/CAN Management/Matrix Cycle Manager/COMP Task - Rx_Vote3_Check/Process_Messages1/Demux message CAN2 and check coherence/UINT8 to UINT16 ==
  In1 : Inport
  In2 : Inport  Port=2
  Bit Shift : hdlsllib/Logic and Bit Operations/Bit Shift  mode=Shift Left Logical  N=8
      settings: SourceProductName=HDL Coder  SourceProductBaseCode=HD
  Cast1 : DataTypeConversion  OutDataTypeStr=uint16
  Cast4 : DataTypeConversion  OutDataTypeStr=uint16
  Sum1 : Sum
  Out1 : Outport
  wires:
  Cast4/1 -> Sum1/1
  Sum1/1 -> Out1/1
  In2/1 -> Cast1/1
  Cast1/1 -> Bit Shift/1
  Bit Shift/1 -> Sum1/2
  In1/1 -> Cast4/1

== stateflow chart HANcoder_E407_GTSync_v5/HANcoder STM32 Target - E407-STM32 algorithm/Global Ticks Increment/CAN Management/Chart ==
  state Send_Trigger
    if (Condition)
    send(Trigger_Signal)
    end
  (default) -> Send_Trigger
  data: Condition input
  events: Trigger_Signal output FUNCTION_CALL_EVENT

== stateflow chart HANcoder_E407_GTSync_v5/HANcoder STM32 Target - E407-STM32 algorithm/Global Ticks Increment/CAN Management/Chart1 ==
  state Send_Trigger
    if (Condition)
    send(Trigger_Signal)
    end
  (default) -> Send_Trigger
  data: Condition input
  events: Trigger_Signal output FUNCTION_CALL_EVENT

== stateflow chart HANcoder_E407_GTSync_v5/HANcoder STM32 Target - E407-STM32 algorithm/Global Ticks Increment/CAN Management/Chart2 ==
  state Send_Trigger
    if (Condition)
    send(Trigger_Signal)
    end
  (default) -> Send_Trigger
  data: Condition input
  events: Trigger_Signal output FUNCTION_CALL_EVENT

== stateflow chart HANcoder_E407_GTSync_v5/HANcoder STM32 Target - E407-STM32 algorithm/Global Ticks Increment/CAN Management/Chart3 ==
  state Send_Trigger
    if (Condition)
    send(Trigger_Signal)
    end
  (default) -> Send_Trigger
  data: Condition input
  events: Trigger_Signal output FUNCTION_CALL_EVENT

== stateflow chart HANcoder_E407_GTSync_v5/HANcoder STM32 Target - E407-STM32 algorithm/Global Ticks Increment/CAN Management/Chart4 ==
  state Send_Trigger
    if (Condition)
    send(Trigger_Signal)
    end
  (default) -> Send_Trigger
  data: Condition input
  events: Trigger_Signal output FUNCTION_CALL_EVENT

== stateflow chart HANcoder_E407_GTSync_v5/HANcoder STM32 Target - E407-STM32 algorithm/Global Ticks Increment/Local Time generation/Chart ==
  state Send_Trigger
    if (Condition)
    send(Trigger_Signal)
    end
  (default) -> Send_Trigger
  data: Condition input
  events: Trigger_Signal output FUNCTION_CALL_EVENT
